simulink model "Force_InnerPosition"  (R2020a)
settings: Solver=VariableStepAuto  StartTime=0.0  StopTime=1  RelTol=1e-3
undefined symbols (not defined in the file): g, KD, KFI, KFP, KP, Md, PI_ctrl
libraries: vrlib x1
settings Model: Creator=Sebastiano  LastModifiedBy=Sebastiano

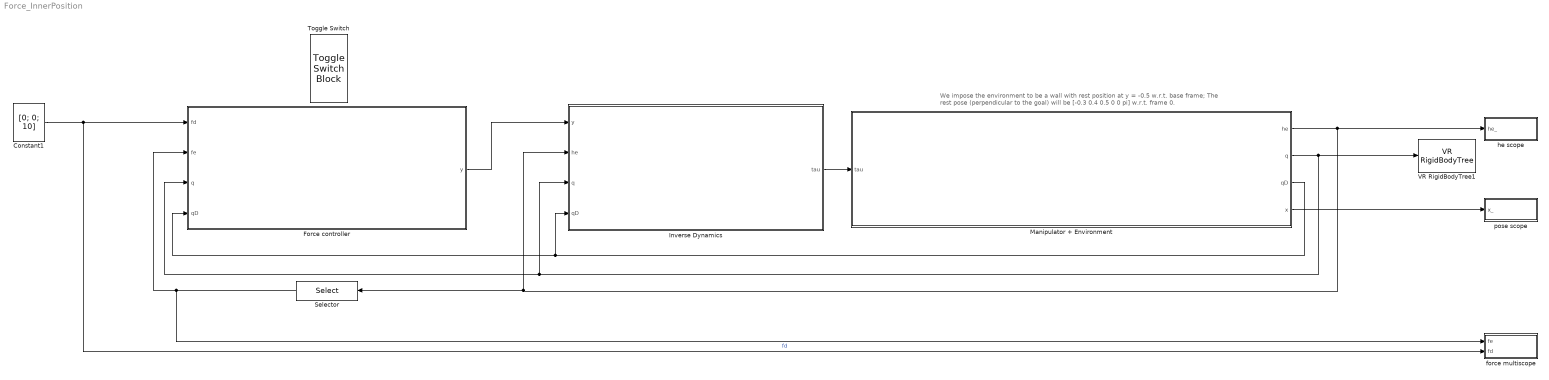
== system Force_InnerPosition ==
  note: We impose the environment to be a wall with rest position at y = -0.5 w.r.t. base frame;
      | The rest pose (perpendicular to the goal) will be [-0.3 0.4 0.5 0 0 pi] w.r.t. frame 0.
  Constant1 : Constant  Value=[0; 0; 10]  VectorParams1D=off
  Force controller : Subsystem
  Inverse Dynamics : Subsystem
  Manipulator + Environment : Subsystem
  Selector : Selector  InputPortWidth=6  IndexOptions=Starting index (dialog)  Indices=1  OutputSizes=3
  Toggle Switch : ToggleSwitchBlock  LabelPosition=Hide
      settings: Values={{'Use PI-action', 'Use P-action'}, [1 0]}
  VR RigidBodyTree1 : vrlib/VR RigidBodyTree  RBT=robot  useRBT=on  Ts=-1  ForceViewerOpen=on
      settings: SourceProductBaseCode=SL
  force multiscope : Subsystem
  he scope : Subsystem
  pose scope : Subsystem
  wires:
  Manipulator + Environment/1(he) -> he scope/1(he_), Selector/1, Inverse Dynamics/2(he)
  Constant1/1 -> force multiscope/2(fd), Force controller/1(fd)  "fd"
  Manipulator + Environment/4(x) -> pose scope/1(x_)
  Manipulator + Environment/3(qD) -> Inverse Dynamics/4(qD), Force controller/4(qD)
  Manipulator + Environment/2(q) -> VR RigidBodyTree1/1, Inverse Dynamics/3(q), Force controller/3(q)
  Force controller/1(y) -> Inverse Dynamics/1(y)
  Selector/1 -> Force controller/2(fe), force multiscope/1(fe)
  Inverse Dynamics/1(tau) -> Manipulator + Environment/1(tau)

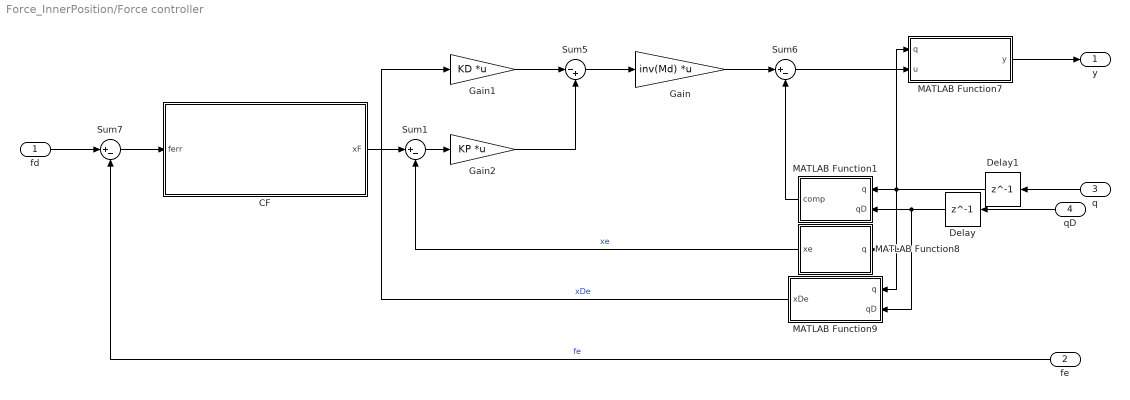
== system Force_InnerPosition/Force controller ==
  fd : Inport
  fe : Inport  Port=2
  q : Inport  Port=3
  qD : Inport  Port=4
  CF : Subsystem
  Delay : Delay  DelayLength=1
  Delay1 : Delay  DelayLength=1
  Gain : Gain  Gain=inv(Md)  Multiplication=Matrix(K*u) (u vector)
  Gain1 : Gain  Gain=KD  Multiplication=Matrix(K*u) (u vector)
  Gain2 : Gain  Gain=KP  Multiplication=Matrix(K*u) (u vector)
  MATLAB Function1 : MATLAB Function  TreatAsAtomicUnit=on
  MATLAB Function7 : MATLAB Function  TreatAsAtomicUnit=on
  MATLAB Function8 : MATLAB Function  TreatAsAtomicUnit=on
  MATLAB Function9 : MATLAB Function  TreatAsAtomicUnit=on
  Sum1 : Sum  Inputs=|+-
  Sum5 : Sum  Inputs=|-+
  Sum6 : Sum  Inputs=|+-
  Sum7 : Sum  Inputs=|+-
  y : Outport
  wires:
  fd/1 -> Sum7/1
  Sum1/1 -> Gain2/1
  MATLAB Function7/1(y) -> y/1
  Gain/1 -> Sum6/1
  MATLAB Function9/1(xDe) -> Gain1/1  "xDe"
  Gain1/1 -> Sum5/1
  fe/1 -> Sum7/2  "fe"
  Sum5/1 -> Gain/1
  MATLAB Function1/1(comp) -> Sum6/2
  Sum6/1 -> MATLAB Function7/2(u)
  Gain2/1 -> Sum5/2
  q/1 -> Delay1/1
  qD/1 -> Delay/1
  MATLAB Function8/1(xe) -> Sum1/2  "xe"
  Sum7/1 -> CF/1(ferr)
  CF/1(xF) -> Sum1/1
  Delay/1 -> MATLAB Function9/2(qD), MATLAB Function1/2(qD)
  Delay1/1 -> MATLAB Function7/1(q), MATLAB Function9/1(q), MATLAB Function8/1(q), MATLAB Function1/1(q)

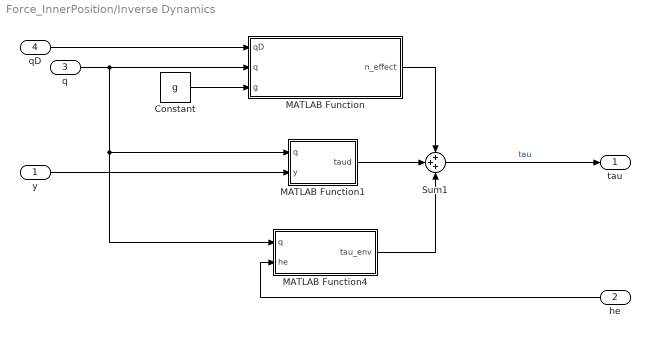
== system Force_InnerPosition/Inverse Dynamics ==
  y : Inport
  he : Inport  Port=2
  q : Inport  Port=3
  qD : Inport  Port=4
  Constant : Constant  Value=g
  MATLAB Function : MATLAB Function  TreatAsAtomicUnit=on
  MATLAB Function1 : MATLAB Function  TreatAsAtomicUnit=on
  MATLAB Function4 : MATLAB Function  TreatAsAtomicUnit=on
  Sum1 : Sum  Inputs=+++
  tau : Outport
  wires:
  qD/1 -> MATLAB Function/1(qD)
  MATLAB Function/1(n_effect) -> Sum1/1
  MATLAB Function1/1(taud) -> Sum1/2
  q/1 -> MATLAB Function/2(q), MATLAB Function4/1(q), MATLAB Function1/1(q)
  Constant/1 -> MATLAB Function/3(g)
  y/1 -> MATLAB Function1/2(y)
  Sum1/1 -> tau/1  "tau"
  MATLAB Function4/1(tau_env) -> Sum1/3
  he/1 -> MATLAB Function4/2(he)

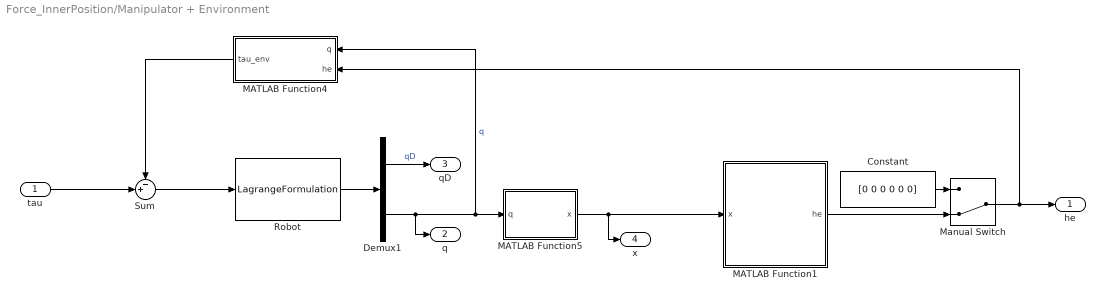
== system Force_InnerPosition/Manipulator + Environment ==
  tau : Inport
  Constant : Constant  Value=[0 0 0 0 0 0]
  Demux1 : Demux  Outputs=[3, 3]
  MATLAB Function1 : MATLAB Function  TreatAsAtomicUnit=on
  MATLAB Function4 : MATLAB Function  TreatAsAtomicUnit=on
  MATLAB Function5 : MATLAB Function  TreatAsAtomicUnit=on
  Manual Switch : ManualSwitch  CurrentSetting=0
  Robot : S-Function  FunctionName=LagrangeFormulation  Parameters=g  SFunctionDeploymentMode=off  EnableBusSupport=off
  Sum : Sum  Inputs=-+|
  he : Outport
  q : Outport  Port=2
  qD : Outport  Port=3
  x : Outport  Port=4
  wires:
  Sum/1 -> Robot/1
  MATLAB Function1/1(he) -> Manual Switch/2
  Robot/1 -> Demux1/1
  MATLAB Function4/1(tau_env) -> Sum/1
  MATLAB Function5/1(x) -> x/1, MATLAB Function1/1(x)
  Constant/1 -> Manual Switch/1
  Manual Switch/1 -> MATLAB Function4/2(he), he/1
  Demux1/2 -> MATLAB Function4/1(q), MATLAB Function5/1(q), q/1  "q"
  tau/1 -> Sum/2
  Demux1/1 -> qD/1  "qD"

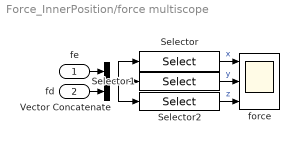
== system Force_InnerPosition/force multiscope ==
  fe : Inport
  fd : Inport  Port=2
  Selector : Selector  InputPortWidth=6  IndexOptions=Index vector (dialog)  Indices=[1 4]  OutputSizes=6
  Selector1 : Selector  InputPortWidth=6  IndexOptions=Index vector (dialog)  Indices=[2 5]  OutputSizes=6
  Selector2 : Selector  InputPortWidth=6  IndexOptions=Index vector (dialog)  Indices=[3 6]  OutputSizes=6
  Vector Concatenate : Concatenate  ConcatenateDimension=2
  force : Scope  NumInputPorts=3
  wires:
  fe/1 -> Vector Concatenate/1
  fd/1 -> Vector Concatenate/2
  Selector1/1 -> force/2  "y"
  Selector/1 -> force/1  "x"
  Vector Concatenate/1 -> Selector2/1, Selector/1, Selector1/1
  Selector2/1 -> force/3  "z"

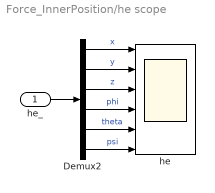
== system Force_InnerPosition/he scope ==
  he_ : Inport
  Demux2 : Demux  Outputs=[1, 1, 1, 1, 1, 1]
  he : Scope  NumInputPorts=6
  wires:
  Demux2/4 -> he/4  "phi"
  Demux2/3 -> he/3  "z"
  Demux2/6 -> he/6  "psi"
  Demux2/5 -> he/5  "theta"
  Demux2/1 -> he/1  "x"
  he_/1 -> Demux2/1
  Demux2/2 -> he/2  "y"

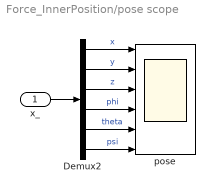
== system Force_InnerPosition/pose scope ==
  x_ : Inport
  Demux2 : Demux  Outputs=[1, 1, 1, 1, 1, 1]
  pose : Scope  NumInputPorts=6
  wires:
  Demux2/4 -> pose/4  "phi"
  Demux2/3 -> pose/3  "z"
  Demux2/6 -> pose/6  "psi"
  Demux2/5 -> pose/5  "theta"
  Demux2/1 -> pose/1  "x"
  x_/1 -> Demux2/1
  Demux2/2 -> pose/2  "y"

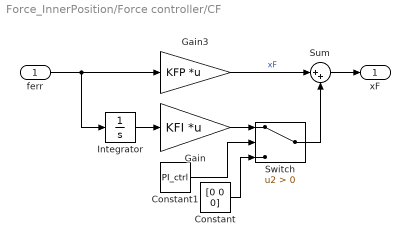
== system Force_InnerPosition/Force controller/CF ==
  ferr : Inport
  Constant : Constant  Value=[0 0 0]
  Constant1 : Constant  Value=PI_ctrl
  Gain : Gain  Gain=KFI  Multiplication=Matrix(K*u) (u vector)
  Gain3 : Gain  Gain=KFP  Multiplication=Matrix(K*u) (u vector)
  Integrator : Integrator
  Sum : Sum  Inputs=|++
  Switch : Switch  Criteria=u2 > Threshold
  xF : Outport
  wires:
  ferr/1 -> Integrator/1, Gain3/1
  Gain3/1 -> Sum/1  "xF"
  Sum/1 -> xF/1
  Gain/1 -> Switch/1
  Switch/1 -> Sum/2
  Integrator/1 -> Gain/1
  Constant/1 -> Switch/3
  Constant1/1 -> Switch/2

== matlab function Force_InnerPosition/Force controller/MATLAB Function7 ==
  data: q input; u input; y output
function y = Jpinv(q, u)

J = Jacobian(q);
Jp = J(1:3,:);
y =  pinv(Jp) * u;

== matlab function Force_InnerPosition/Force controller/MATLAB Function1 ==
  data: q input; comp output; qD input
function comp = JpD(q, qD)

t1 = q(1);
t2 = q(2);
d3 = q(3);

Dt1 = qD(1);
Dt2 = qD(2);
Dd3 = qD(3);

JpD = [[ - 2/5*Dt1*cos(t1) - 3/10*cos(t1 + t2)*(Dt1 + Dt2), -3/10*cos(t1 + t2)*(Dt1 + Dt2), 0];
       [ - 3/10*sin(t1 + t2)*(Dt1 + Dt2) - 2/5*Dt1*sin(t1), -3/10*sin(t1 + t2)*(Dt1 + Dt2), 0];
       [                                                 0,                              0, 0]];

comp = JpD*qD;

== matlab function Force_InnerPosition/Inverse Dynamics/MATLAB Function ==
  data: qD input; q input; n_effect output; g input
function n_effect = n(qD, q, g)

n_effect = C_Lagrangian(q, qD)*qD + G_Lagrangian(q, g);

== matlab function Force_InnerPosition/Inverse Dynamics/MATLAB Function1 ==
  data: q input; taud output; y input
function taud = B(q, y)

taud = B_Lagrangian(q)*y;

== matlab function Force_InnerPosition/Inverse Dynamics/MATLAB Function4 ==
  data: q input; he input; tau_env output
function tau_env = J(q, he)

tau_env = Jacobian(q)' * he;

== matlab function Force_InnerPosition/Force controller/MATLAB Function8 ==
  data: q input; xe output
function xe = Kp(q)

t1 = q(1);
t2 = q(2);
d3 = q(3);

K = [[ cos(t1 + t2), -sin(t1 + t2), 0, (3*cos(t1 + t2))/10 + (2*cos(t1))/5]
     [ sin(t1 + t2),  cos(t1 + t2), 0, (3*sin(t1 + t2))/10 + (2*sin(t1))/5]
     [            0,             0, 1,                            d3 + 2/5]
     [            0,             0, 0,                                   1]];

pos = K(1:3, 4);

xe = [pos];

== matlab function Force_InnerPosition/Force controller/MATLAB Function9 ==
  data: q input; xDe output; qD input
function xDe = Jp(q, qD)

J = Jacobian(q);
Jp = J(1:3,:);
xDe = Jp * qD;

== matlab function Force_InnerPosition/Manipulator + Environment/MATLAB Function1 ==
  data: x input; he output
function he = environment(x)

% environment params
K = diag([15 15 15 0.1 0.1 0.1]);    % stiffness
wall = 0.5; % constraint position w.r.t. frame 0 (it's y=-0.5 w.r.t. base frame)

if x(3) >= wall  % check is done in frame 0
    % touching the environment! constrained motion
    % set up the rest position frame
    % (basically, same orientation as ee but position is the contact point at the wall)
    xr = x;
    xr(3) = wall;
    % calculate the forces
    dx_re = x - xr;
    he = K * dx_re;
else
    % free motion
    he = zeros(6,1);
end

he = reshape(he,[6 1]);

== matlab function Force_InnerPosition/Manipulator + Environment/MATLAB Function4 ==
  data: q input; he input; tau_env output
function tau_env = J(q, he)

tau_env = Jacobian(q)' * he;

== matlab function Force_InnerPosition/Manipulator + Environment/MATLAB Function5 ==
  data: q input; x output
function x = K(q)

t1 = q(1);
t2 = q(2);
d3 = q(3);

K = [[ cos(t1 + t2), -sin(t1 + t2), 0, (3*cos(t1 + t2))/10 + (2*cos(t1))/5]
     [ sin(t1 + t2),  cos(t1 + t2), 0, (3*sin(t1 + t2))/10 + (2*sin(t1))/5]
     [            0,             0, 1,                            d3 + 2/5]
     [            0,             0, 0,                                   1]];

pos = K(1:3, 4);
ori = rotm2eul(K(1:3,1:3), 'ZYZ')';

x = [pos; ori];
